simulink library "TalariaApiBuffer"  (R2022b)
settings: Solver=VariableStepAuto  StartTime=0.0  StopTime=10.0  RelTol=1e-3
libraries: HandyTextFile x2
settings Model: Creator=kl13806  LastModifiedBy=kl13806
settings SolverCC: AlgebraicLoopSolver=TrustRegion
settings DebuggingCC: UnconnectedInputMsg=warning  UnconnectedOutputMsg=warning  UnconnectedLineMsg=warning  SFMachineParentedDataDiag=warning  ArithmeticOperatorsInVariantConditions=warning
settings ModelReferenceCC: EnableRefExpFcnMdlSchedulingChecks=on
settings SFSimCC: CustomCodeUndefinedFunction=UseInterfaceOnly
settings RTWCC: DLArmComputeVersion=19.05

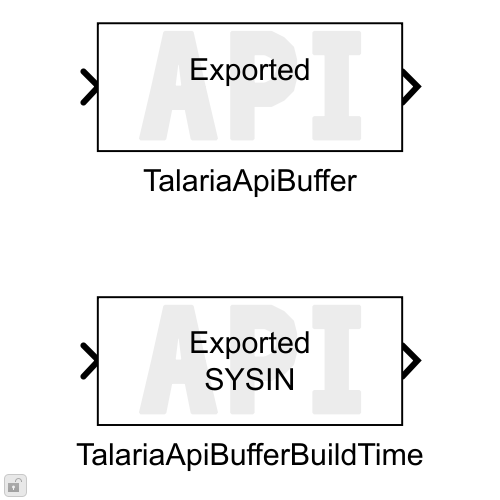
[thumbnail: Simulink's stored preview of the top-level diagram]
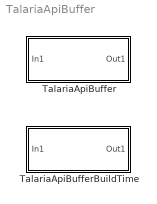
== system TalariaApiBuffer ==
  TalariaApiBuffer : Subsystem  mask(Talaria API Buffer){MaskSignalName=, BufferAccess=Exported: storage defined in generated code, TriggerInit=[]}
      mask prompts: MaskSignalName "Signal Buffer Name:"; TriggerInit "Hidden: MoveFcn redraw"
      mask help: This block sets a signal line's name and storage class in generated source code for the TalariaAPI.h header file.
      mask init:
      | [ok] = TalariaApiBufferMask.Init(gcbh,MaskSignalName,BufferAccess);
      settings: MoveFcn=TalariaApiBufferMask.CB_TriggerInit(gcbh);
      mask Help: The Signal Name you provide is a starting point for the symbol defined in generated code. However, if more than one line in the same model shares the same name, the generated code will mangle unique prefix/suffix elements to each code symbol to ensure uniqueness.
      mask TypeOptions BufferAccess: Exported: storage defined in generated code | Imported: storage defined externally | Imported pointer: storage allocated externally | Exported pointer: storage allocated externally
      mask Callback TriggerInit: TalariaApiBufferMask.CB_TriggerInit(gcbh);
      mask DialogControl ErrorContainer Prompt: Error Messages
      mask Display:
      | [path,w,h] = IconTalariaApiBufferMask();
      | 
      | % retrieve the block's pixel size
      | pos = get(gcbh,'position');
      | bw = pos(3) - pos(1);
      | bh = pos(4) - pos(2);
      | 
      | % Draw centered icon
      | xAdj = bw/2 - w/2;
      | yAdj = bh/2 - h/2;
      | for i=1:length(path)
      |     if (path(i).rgb(1) >= 0)
      |         patch(path(i).x+xAdj, path(i).y+yAdj, path(i).rgb);
      |     end
      |     if (path(i).stroke(1) >= 0)
      |         plot(path(i).x+xAdj, path(i).y+yAdj);
      |     end
      | end
      | 
      | % show text or an X
      | if (exist('ok','var') && ok)
      |    access = strtok(get_param(gcbh,'BufferAccess'),':');
      |    text(bw*0.5, bh*0.5, [access newline MaskSignalName], 'horizontalAlignment', 'center');
      |    patch(0,0,[1 1 1]);
      |    patch(bw,bh,[1 1 1]);
      | else
      |    tx=bw*0.03;
      |    ty=bh*0.03;
      |    patch([0 tx bw bw-tx], [ty 0 bh-ty bh], [1 0 0]);
      |    patch([0 bw-tx bw tx], [bh-ty 0 ty bh], [1 0 0]);
      | end
  TalariaApiBufferBuildTime : Subsystem  mask(Talaria API Buffer){Config=[], TriggerInit=[30 114 130 156]}
      mask prompts: Config "TalariaApiBufferBuildTimeConfig"; TriggerInit "Hidden: MoveFcn redraw"
      mask help:
      | This block sets a signal line's name and storage class in generated source code for the TalariaAPI.h header file.
      | This version of the block receives all settings from a build-time configuration classdef.
      mask init:
      | blkh=gcbh;
      | Config=BTConfig.Assert(blkh,Config);
      | [ok] = TalariaApiBufferBTMask.Init(blkh,Config.BufferName,Config.AccessType);
      | Config.Validate();
      settings: MoveFcn=TalariaApiBufferMask.CB_TriggerInit(gcbh);
      mask Help: The Signal Name you provide is a starting point for the symbol defined in generated code. However, if more than one line in the same model shares the same name, the generated code will mangle unique prefix/suffix elements to each code symbol to ensure uniqueness.
      mask Callback TriggerInit: TalariaApiBufferMask.CB_TriggerInit(gcbh);
      mask DialogControl ErrorContainer Prompt: Error Messages
      mask Display:
      | [path,w,h] = IconTalariaApiBufferMask();
      | 
      | % retrieve the block's pixel size
      | pos = get(gcbh,'position');
      | bw = pos(3) - pos(1);
      | bh = pos(4) - pos(2);
      | 
      | % Draw centered icon
      | xAdj = bw/2 - w/2;
      | yAdj = bh/2 - h/2;
      | for i=1:length(path)
      |     if (path(i).rgb(1) >= 0)
      |         patch(path(i).x+xAdj, path(i).y+yAdj, path(i).rgb);
      |     end
      |     if (path(i).stroke(1) >= 0)
      |         plot(path(i).x+xAdj, path(i).y+yAdj);
      |     end
      | end
      | 
      | % show text or an X
      | if (exist('ok','var') && ok)
      |     access = TalariaApiBufferBTMask.GetAccessDescription(Config.AccessType);
      | 	text(bw*0.5, bh*0.5, [access newline Config.BufferName], 'horizontalAlignment', 'center');
      | 	patch(0,0,[1 1 1]);
      | 	patch(bw,bh,[1 1 1]);
      | else
      | 	tx=bw*0.03;
      | 	ty=bh*0.03;
      | 	patch([0 tx bw bw-tx], [ty 0 bh-ty bh], [1 0 0]);
      | 	patch([0 bw-tx bw tx], [bh-ty 0 ty bh], [1 0 0]);
      | end

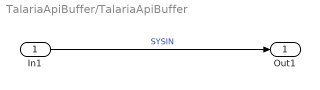
== system TalariaApiBuffer/TalariaApiBuffer ==
  In1 : Inport
  Out1 : Outport  VectorParamsAs1DForOutWhenUnconnected=off
  wires:
  In1/1 -> Out1/1  "SYSIN"

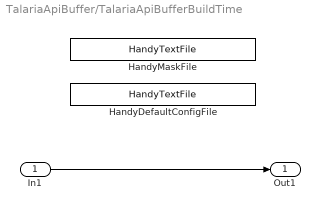
== system TalariaApiBuffer/TalariaApiBufferBuildTime ==
  In1 : Inport
  HandyDefaultConfigFile : HandyTextFile/HandyTextFile  TemplateSource=Config  FileSuffix=Config.m  OpenDialogOnLoad=off  UseThisBlockName=off  TheDefaultText=|  ShowInLibBrowser=on
      | classdef $(PREFIX)$(SUFFIX)
      | % $(FILENAME) Class definition to contain build-time configuration for $(PREFIX)
      | % Usage:
      | %    aConfig = $(PREFIX)$(SUFFIX)
      | %
      | 
      | %   Copyright 2020 Bose Corporation
      | 
      |   properties
      |     % Properties use this syntax:
      |     %    PropertyName size class {validation functions} = DefaultValue
      |     % About Build-Time Configuration: https://wiki.bose.com/x/dqPoB
      | 
      |     % Delete these examples:
      |     %Gain = 0.5
      |     %Theta = sin(pi/12)
      |     %MyDoubleArray (1,7) double {mustBeFinite} = [1 2 3 4 5 6 7]
      |     %LeftConfig (1,1) SubBlockConfig
      |     %RightConfig (1,1) SubBlockConfig
      | 
      |   end
      | end
      settings: SourceProductName=Bose Talaria
  HandyMaskFile : HandyTextFile/HandyTextFile  TemplateSource=Mask  FileSuffix=Mask.m  OpenDialogOnLoad=off  UseThisBlockName=off  TheDefaultText=|  ShowInLibBrowser=on
      | classdef $(PREFIX)$(SUFFIX)
      | % $(FILENAME): $(SUFFIX) logic for the $(PREFIX) block
      | 
      | %   Copyright 2020 Bose Corporation
      | 
      |     methods (Static)
      |         function DoInit(H)
      |         end
      |     end
      | end
      settings: SourceProductName=Bose Talaria
  Out1 : Outport  VectorParamsAs1DForOutWhenUnconnected=off
  wires:
  In1/1 -> Out1/1
